simulink model "PRAVEENKUMARCLO"  (R2015b)
settings: Solver=VariableStepAuto  StartTime=0.0  StopTime=10  RelTol=1e-3
libraries: powerlib x28, powerlib_meascontrol x4, electricdrivelib x1, simulink x1
settings Model: Creator=SPIRO  LastModifiedBy=SPIRO

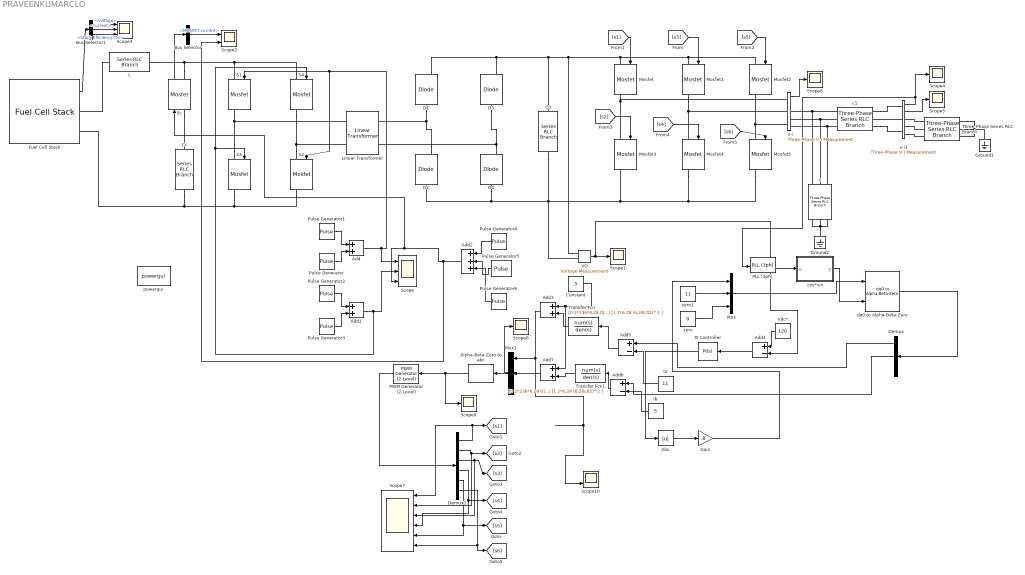
== system PRAVEENKUMARCLO ==
  Abs : Abs
  Add{,1,3,7} (4 alike) : Sum
  Add2 : Sum  Inputs=+++
  Add4 : Sum  Inputs=+-
  Add5 : Sum  Inputs=+-
  Add6 : Sum  Inputs=+-
  Alpha-Beta-Zero to abc : powerlib_meascontrol/Transformations/Alpha-Beta-Zero to abc
  Bus Selector : BusSelector  OutputSignals=MOSFET current
  Bus Selector1 : BusSelector  OutputSignals=Voltage,Current,Stack Efficiency (%)
  C0 : powerlib/Elements/Series RLC Branch  LConnTagsString=__new0  RConnTagsString=__new0  BranchType=C  Resistance=1  Inductance=1e-3  SetiL0=off  InitialCurrent=0  Capacitance=100e-6  Setx0=off  InitialVoltage=0  Measurements=None
  Cc : powerlib/Elements/Series RLC Branch  LConnTagsString=__new0  RConnTagsString=__new0  BranchType=C  Resistance=1  Inductance=1e-3  SetiL0=off  InitialCurrent=0  Capacitance=1000e-6  Setx0=off  InitialVoltage=0  Measurements=None
  Constant : Constant  Value=.5
  D{1..4} (4 alike) : powerlib/Power Electronics/Diode  Ron=0.001  Lon=0  Vf=0.8  IC=0  UseSnubber=off  Rs=500  Cs=250e-9  Measurements=on
  Demux : Demux  Outputs=3
  Demux1 : Demux  Outputs=6
  Fuel Cell Stack : electricdrivelib/Extra Sources/Fuel Cell Stack  PresetModel=No (User-Defined)  FcType=0  Detailed=Detailed  Eoc="[65  63]"  NomVI="[133.3            45]"  EndVI="[225   37]"  Nc=65  n=55  TOp=65  AirFr=300  SuppPress="[1.5           1]"  Comp="[99.95           21            1]"  SignX=off  SignY=off  FlowRateH2=off  FlowRateAir=off  SystemTemp=off  SystemPH2=off  SystemPAir=off  FCDyn=off  FC_tau=1  Peak_O2=80  V_Under=10
  Gain : Gain  Gain=.8
  Ground1 : powerlib/Elements/Ground  LConnTagsString=a
  Ground2 : powerlib/Elements/Ground  LConnTagsString=a
  Ia : Constant  Value=11
  Ib : Constant  Value=5
  L : powerlib/Elements/Series RLC Branch  LConnTagsString=__new0  RConnTagsString=__new0  BranchType=L  Resistance=1  Inductance=.90e-3  SetiL0=off  InitialCurrent=0  Capacitance=1e-6  Setx0=off  InitialVoltage=0  Measurements=None
  Linear Transformer : powerlib/Elements/Linear Transformer  UNITS=pu  NominalPower=[ 25e3 10e3 ]  winding1="[ 1000  0.002  0.08 ]"  winding2="[ 1000  0.002  0.08 ]"  ThreeWindings=off  winding3=[ 315e3 0.002 0.08 ]  RmLm=[ 50 50]  Measurements=None  DataType=off
  Mosfet{,1..5} (6 alike) : powerlib/Power Electronics/Mosfet  Ron=0.1  Lon=0  Rd=0.01  Vfd=0  IC=0  Rs=1e5  Cs=inf  Measurements=on
  Mux : Mux  Inputs=3
  Mux1 : Mux  Inputs=3
  PI Controller : simulink/Continuous/PID Controller  Controller=PI  TimeDomain=Continuous-time  SampleTime=-1  IntegratorMethod=Forward Euler  FilterMethod=Forward Euler  Form=Parallel  UseFilter=on  ControllerParametersSource=internal  P=1  I=1.5  D=0  N=100  InitialConditionSource=internal  InitialConditionForIntegrator=0  InitialConditionForFilter=0  ExternalReset=none  LimitOutput=off  UpperSaturationLimit=inf  LowerSaturationLimit=-inf  LinearizeAsGain=on  AntiWindupMode=none  Kb=1  TrackingMode=off  Kt=1  PParamMin=[]  PParamMax=[]  IParamMin=[]  IParamMax=[]  DParamMin=[]  DParamMax=[]  NParamMin=[]  NParamMax=[]  KbParamMin=[]  KbParamMax=[]  KtParamMin=[]  KtParamMax=[]  POutMin=[]  POutMax=[]  IOutMin=[]  IOutMax=[]  DOutMin=[]  DOutMax=[]  NOutMin=[]  NOutMax=[]  KbOutMin=[]  KbOutMax=[]  KtOutMin=[]  KtOutMax=[]  IntegratorOutMin=[]  IntegratorOutMax=[]  FilterOutMin=[]  FilterOutMax=[]  SumOutMin=[]  SumOutMax=[]  SumI1OutMin=[]  SumI1OutMax=[]  SumI2OutMin=[]  SumI2OutMax=[]  SumI3OutMin=[]  SumI3OutMax=[]  SumDOutMin=[]  SumDOutMax=[]  SaturationOutMin=[]  SaturationOutMax=[]  IntegratorContinuousStateAttributes=''  IntegratorStateMustResolveToSignalObject=off  IntegratorRTWStateStorageClass=Auto  FilterContinuousStateAttributes=''  FilterStateMustResolveToSignalObject=off  FilterRTWStateStorageClass=Auto  DifferentiatorICPrevScaledInput=0  DifferentiatorOutMin=[]  DifferentiatorOutMax=[]
  PLL (3ph) : powerlib_meascontrol/PLL/PLL (3ph)  Fmin=45  Par_Init=[0, 60]  ParK=[180, 3200, 1]  TcD=1e-4  MaxRateChangeFreq=12  FilterCutOffFreq=25  Ts=0  AGC=on
  PWM Generator (2-Level) : powerlib_meascontrol/Pulse & Signal Generators/PWM Generator (2-Level)  ModulatorType=Three-phase bridge (6 pulses)  ModulatorMode=Unsynchronized  Fc=50  Pc=90  nF=27  MinMax="[ -1  1 ]"  SamplingTechnique=Natural  ModulatingSignals=off  m=0.8  Freq=60  Phase=0  Ts=0  ShowCarrierOutport=off
  Pulse Generator : DiscretePulseGenerator  PulseType=Time based  Period=.0002  PulseWidth=(1/2)*100
  Pulse Generator1 : DiscretePulseGenerator  PulseType=Time based  Period=.0002  PulseWidth=(.6/2)*100  PhaseDelay=(1.4/2)*.0002
  Pulse Generator2 : DiscretePulseGenerator  PulseType=Time based  Period=.0002  PulseWidth=(.3/2)*100
  Pulse Generator3 : DiscretePulseGenerator  PulseType=Time based  Period=.0002  PulseWidth=(1/2)*100  PhaseDelay=(.7/2)*.0002
  Pulse Generator4 : DiscretePulseGenerator  PulseType=Time based  Period=.0002  PulseWidth=(.3/2)*100  PhaseDelay=(.35/2)*.0002
  Pulse Generator5 : DiscretePulseGenerator  PulseType=Time based  Period=.0002  PulseWidth=(.3/2)*100  PhaseDelay=(1.05/2)*.0002
  Pulse Generator6 : DiscretePulseGenerator  PulseType=Time based  Period=.0002  PulseWidth=(.3/2)*100  PhaseDelay=(1.7/2)*.0002
  S{1..4} (4 alike) : powerlib/Power Electronics/Mosfet  Ron=0.1  Lon=0  Rd=0.01  Vfd=0  IC=0  Rs=1e5  Cs=inf  Measurements=on
  Sc : powerlib/Power Electronics/Mosfet  Ron=0.01  Lon=0  Rd=0.001  Vfd=0  IC=0  Rs=1e5  Cs=inf  Measurements=on
  Scope : Scope  NumInputPorts=3
  Scope{1,4..6,8..9} (6 alike) : Scope
  Scope10 : Scope  NumInputPorts=2
  Scope2 : Scope  NumInputPorts=2
  Scope3 : Scope  NumInputPorts=3
  Scope7 : Scope  NumInputPorts=6
  Three-Phase Series RLC Branch : powerlib/Elements/Three-Phase Series RLC Branch  LConnTagsString=A|B|C  RConnTagsString=A|B|C  BranchType=R  Resistance=500  Inductance=100e-3  Capacitance=1e-6  Measurements=None
  Transfer Fcn : TransferFcn  Numerator=[0 2*236*6.28 0]  Denominator=[1 2*6.28 (6.28/.02)^2 ]
  Transfer Fcn1 : TransferFcn  Numerator=[0 2*236*6.28 0]  Denominator=[1 2*6.28 (6.28/.02)^2 ]
  VO : powerlib/Measurements/Voltage Measurement  PhasorSimulation=off  OutputType=Complex  PSBequivalent=0
  Vdc* : Constant  Value=120
  c : powerlib/Elements/Three-Phase Series RLC Branch  LConnTagsString=A|B|C  RConnTagsString=A|B|C  BranchType=C  Resistance=10  Inductance=100e-3  Capacitance=9e-6  Measurements=None
  c1 : powerlib/Elements/Three-Phase Series RLC Branch  LConnTagsString=A|B|C  RConnTagsString=A|B|C  BranchType=L  Resistance=10  Inductance=.8  Capacitance=100e-6  Measurements=None
  cos*sin : MATLAB Function  TreatAsAtomicUnit=on
  dq0 to Alpha-Beta-Zero : powerlib_meascontrol/Transformations/dq0 to Alpha-Beta-Zero  Alignment=90 degrees behind phase A axis
  powergui : powerlib/powergui  Priority=1  SimulationMode=Discrete  SolverType=Tustin/Backward Euler (TBE)  SampleTime=50e-6  frequency=60  SPID=off  DisableSnubberDevices=off  DisableRonSwitches=off  DisableVfSwitches=off  SwTol=0  DisplayEquations=off  Interpol=off  ExternalGateDelay=off  methode=off  Ts=10  FunctionMessages=off  echomessages=off  HookPort=off  EnableUseOfTLC=off  x0status=blocks  frequencyindice=0  Pbase=100e6  ErrMax=1e-4  Iterations=50  UnitsV=kV  UnitsW=MW  buscounter=0  RestoreLinks=warning  ResistiveCurrentMeasurement=off  Frange=[0:2:500]  Ylog=off  Xlog=on  ShowGrid=off  save=off  variable=ZData  structure=v  ZoomFFT=off  StartTime=.5  cycles=5  DisplayStyle=1  fundamental=50  FreqAxis=off  MaxFrequency=1000  frequencyindicesteady=1  RmsSteady=1  display=off
  v-i : powerlib/Measurements/Three-Phase V-I Measurement  VoltageMeasurement=phase-to-ground  SetLabelV=off  LabelV=Vabc  Vpu=off  VpuLL=off  CurrentMeasurement=yes  SetLabelI=off  LabelI=Iabc  Ipu=off  Pbase=100e6  Vbase=500e3  OutputType=Complex  PhasorSimulation=off  PSBequivalent=0
  v-i1 : powerlib/Measurements/Three-Phase V-I Measurement  VoltageMeasurement=phase-to-ground  SetLabelV=off  LabelV=Vabc  Vpu=off  VpuLL=off  CurrentMeasurement=yes  SetLabelI=off  LabelI=Iabc  Ipu=off  Pbase=100e6  Vbase=500e3  OutputType=Complex  PhasorSimulation=off  PSBequivalent=0
  zero : Constant  Value=0
  zero1 : Constant  Value=11
  wires:
  Pulse Generator1/1 -> Add/1
  Pulse Generator/1 -> Add/2
  Pulse Generator2/1 -> Add1/1
  Pulse Generator3/1 -> Add1/2
  Pulse Generator4/1 -> Add2/1
  Pulse Generator5/1 -> Add2/2
  Pulse Generator6/1 -> Add2/3
  Add/1 -> S2/1, S1/1, Scope/1
  Add1/1 -> S4/1, S3/1, Scope/2
  Add2/1 -> Scope2/2, Sc/1, Scope/3
  VO/1 -> Add4/2, Scope1/1
  Sc/1 -> Bus Selector/1
  Bus Selector/1 -> Scope2/1  "<MOSFET current>"
  Fuel Cell Stack/1 -> Bus Selector1/1
  Bus Selector1/1 -> Scope3/1  "<Voltage>"
  Bus Selector1/2 -> Scope3/2  "<Current>"
  Bus Selector1/3 -> Scope3/3  "<Stack Efficiency (%)>"
  v-i/1 -> Scope6/1
  v-i1/1 -> Scope4/1, PLL (3ph)/1
  v-i1/2 -> Scope5/1
  PLL (3ph)/2 -> cos*sin/1(u)
  cos*sin/1(y) -> dq0 to Alpha-Beta-Zero/2
  Vdc*/1 -> Add4/1
  Add4/1 -> PI Controller/1
  Mux/1 -> dq0 to Alpha-Beta-Zero/1
  zero1/1 -> Mux/2
  Ia/1 -> Add5/2
  dq0 to Alpha-Beta-Zero/1 -> Demux/1
  Add5/1 -> Transfer Fcn/1
  Ib/1 -> Add6/2
  Add6/1 -> Transfer Fcn1/1
  zero/1 -> Mux/3
  Demux/2 -> Add6/1
  Add7/1 -> Mux1/2
  Constant/1 -> Add3/1, Add7/1
  Transfer Fcn/1 -> Add3/2
  Transfer Fcn1/1 -> Add7/2
  Add3/1 -> Scope10/2, Mux1/1
  Gain/1 -> Mux/1
  Mux1/1 -> Alpha-Beta-Zero to abc/1, Scope8/1
  PI Controller/1 -> Abs/1
  Abs/1 -> Gain/1
  Demux/1 -> Add5/1
  [s3] -> Mosfet1/1
  [s1] -> Mosfet/1
  [s5] -> Mosfet2/1
  [s2] -> Mosfet3/1
  [s4] -> Mosfet4/1
  [s6] -> Mosfet5/1
  Demux1/1 -> Scope7/1, [s1]
  Demux1/2 -> Scope7/2, [s2]
  Demux1/3 -> Scope7/3, [s3]
  Demux1/4 -> Scope7/4, [s4]
  Demux1/6 -> Scope7/6, [s6]
  PWM Generator (2-Level)/1 -> Demux1/1
  Alpha-Beta-Zero to abc/1 -> Scope9/1, PWM Generator (2-Level)/1
  Demux1/5 -> Scope7/5, [s5]
  ? -> Mux1/3, Scope10/1
  connections:
  Sc/RConn1 -- L/RConn1 -- S1/LConn1 -- S4/LConn1
  S3/RConn1 -- S2/RConn1 -- Cc/RConn1 -- Fuel Cell Stack/RConn2
  S3/LConn1 -- S1/RConn1 -- Linear Transformer/LConn1
  S2/LConn1 -- S4/RConn1 -- Linear Transformer/LConn2
  D2/RConn1 -- D1/LConn1 -- Linear Transformer/RConn1
  D4/RConn1 -- D3/LConn1 -- Linear Transformer/RConn2
  Mosfet1/LConn1 -- Mosfet2/LConn1 -- C0/LConn1 -- D3/RConn1 -- D1/RConn1 -- VO/LConn1 -- Mosfet/LConn1
  D2/LConn1 -- D4/LConn1 -- VO/LConn2 -- C0/RConn1 -- Mosfet3/RConn1 -- Mosfet4/RConn1 -- Mosfet5/RConn1
  v-i/LConn3 -- Mosfet5/LConn1 -- Mosfet2/RConn1
  v-i/LConn2 -- Mosfet4/LConn1 -- Mosfet1/RConn1
  Mosfet3/LConn1 -- v-i/LConn1 -- Mosfet/RConn1
  Three-Phase Series RLC Branch/RConn1 -- Three-Phase Series RLC Branch/RConn3 -- Three-Phase Series RLC Branch/RConn2 -- Ground1/LConn1
  c/RConn3 -- c/RConn1 -- Ground2/LConn1 -- c/RConn2
  v-i/RConn1 -- c1/RConn1 -- c/LConn1
  v-i/RConn2 -- c1/RConn2 -- c/LConn2
  c/LConn3 -- c1/RConn3 -- v-i/RConn3
  L/LConn1 -- Fuel Cell Stack/RConn1
  Three-Phase Series RLC Branch/LConn2 -- v-i1/RConn2
  Three-Phase Series RLC Branch/LConn3 -- v-i1/RConn3
  Sc/LConn1 -- Cc/LConn1
  c1/LConn1 -- v-i1/LConn1
  c1/LConn3 -- v-i1/LConn3
  v-i1/LConn2 -- c1/LConn2
  Three-Phase Series RLC Branch/LConn1 -- v-i1/RConn1

== matlab function PRAVEENKUMARCLO/cos*sin ==
  data: u input; y output
function y = fcn(u)
%#codegen

y = sin(u);
